simulink model "motorcontrol"  (R2013a)
settings: Solver=ode45  StartTime=0.0  StopTime=10.0  RelTol=1e-3
settings Model: Creator=jdelange  LastModifiedBy=jdelange

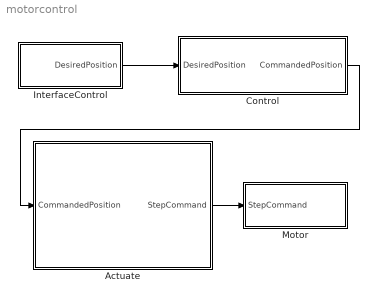
== system motorcontrol ==
  Actuate : Subsystem
  Control : Subsystem
  InterfaceControl : Subsystem
  Motor : Subsystem
  wires:
  InterfaceControl/1(DesiredPosition) -> Control/1(DesiredPosition)
  Control/1(CommandedPosition) -> Actuate/1(CommandedPosition)
  Actuate/1(StepCommand) -> Motor/1(StepCommand)

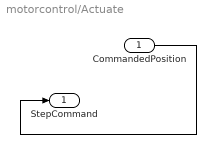
== system motorcontrol/Actuate ==
  CommandedPosition : Inport
  StepCommand : Outport
  wires:
  CommandedPosition/1 -> StepCommand/1

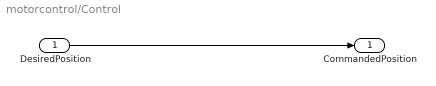
== system motorcontrol/Control ==
  DesiredPosition : Inport
  CommandedPosition : Outport
  wires:
  DesiredPosition/1 -> CommandedPosition/1

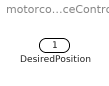
== system motorcontrol/InterfaceControl ==
  DesiredPosition : Outport

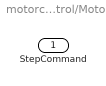
== system motorcontrol/Motor ==
  StepCommand : Inport
